simulink model "MultiTask"  (R2014a)
settings: Solver=FixedStepDiscrete  StartTime=0.0  StopTime=inf  FixedStep=0.005  RelTol=1e-3  SampleTimeConstraint=Specified
libraries: simulink x2, etargetslib x2, dspnetwork x2
settings Model: Creator=ses  LastModifiedBy=ses
settings OptimizationCC: OptimizeModelRefInitCode=on  LifeSpan=Inf  MaxStackSize=64
settings HardwareCC: ProdLargestAtomicInteger=Long  ProdLargestAtomicFloat=Double  ProdEndianess=LittleEndian  ProdHWDeviceType=ARM Compatible->ARM Cortex
settings RTWCC: SystemTargetFile=ert_linux.tlc  MakeCommand=make_rtw CC=arm-linux-gnueabihf-gcc  TemplateMakefile=ert_linux.tmf  Description=Linux Embedded Coder  ProcessScript=ert_linux_make_rtw_hook
settings CodeAppCC: IgnoreCustomStorageClasses=off
settings STFCustomTargetCC: ModelReferenceCompliant=off  ConcurrentExecutionCompliant=off  GeneratePreprocessorConditionals=Use local settings  CombineOutputUpdateFcns=on  ERTCustomFileBanners=on  SupportContinuousTime=off  SupportNonInlinedSFcns=off  MATLABClassNameForMDSCustomization=Simulink.SoftwareTarget.ERTCustomization  GRTInterface=off  SystemTargetFile=ert_linux.tlc
settings ERTTargetCC: GenerateSampleERTMain=off  ModelReferenceCompliant=off  ERTCustomFileTemplate=ert_linux_file_process.tlc

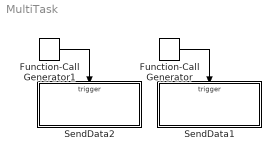
== system MultiTask ==
  Function-Call Generator : simulink/Ports & Subsystems/Function-Call Generator  sample_time=0.005  numberOfIterations=1
  Function-Call Generator1 : simulink/Ports & Subsystems/Function-Call Generator  sample_time=0.01  numberOfIterations=1
  SendData1 : Subsystem  TreatAsAtomicUnit=on
  SendData2 : Subsystem  TreatAsAtomicUnit=on
  wires:
  Function-Call Generator/1 -> SendData1/Trigger
  Function-Call Generator1/1 -> SendData2/Trigger

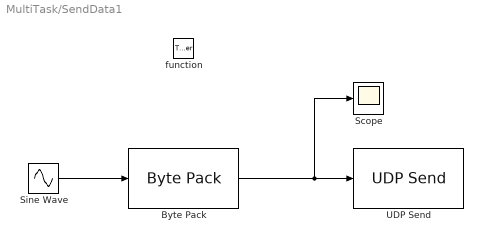
== system MultiTask/SendData1 ==
  function : TriggerPort  TriggerType=function-call  SampleTime=0.005
  Byte Pack : etargetslib/Byte Pack  datatypes={'double'}  byteAlign=1
  Scope : Scope
  Sine Wave : Sin
  UDP Send : dspnetwork/UDP Send  remoteURL='192.168.0.11'  remotePort=5000  localURL='0.0.0.0'  localPortSource=Automatically determine  localPort=51000  sampletime=-1  blockPlatform=LINUX  separateLengthPort=0
  wires:
  Byte Pack/1 -> Scope/1, UDP Send/1
  Sine Wave/1 -> Byte Pack/1

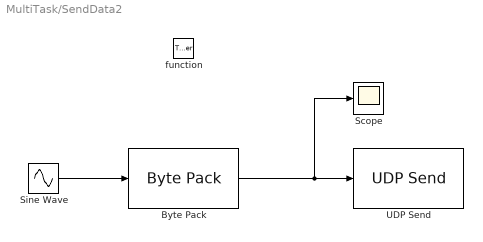
== system MultiTask/SendData2 ==
  function : TriggerPort  TriggerType=function-call  SampleTime=0.005
  Byte Pack : etargetslib/Byte Pack  datatypes={'double'}  byteAlign=1
  Scope : Scope
  Sine Wave : Sin
  UDP Send : dspnetwork/UDP Send  remoteURL='192.168.0.11'  remotePort=5100  localURL='0.0.0.0'  localPortSource=Automatically determine  localPort=51000  sampletime=-1  blockPlatform=LINUX  separateLengthPort=0
  wires:
  Sine Wave/1 -> Byte Pack/1
  Byte Pack/1 -> UDP Send/1, Scope/1
